simulink model "Tra_Add"  (R2016b)
settings: configuration reference "CodeGenConfigSet" (kept outside this file)
values from neighbouring files (symbols this model uses):
  Tra_bCanAirCanPtd_C = Calibration.Parameter    [init_Tra_Add.m]    (also in init_Tra_Add_SIL.m = Simulink.Parameter)
  Tra_bCanClntCanPtd_C = Calibration.Parameter    [init_Tra_Add.m]    (also in init_Tra_Add_SIL.m = Simulink.Parameter)
  Tra_rClgDem_C = Calibration.Parameter    [init_Tra_Add.m]    (also in init_Tra_Add_SIL.m = Simulink.Parameter)
  Tra_tClntDes_C = Calibration.Parameter    [init_Tra_Add.m]    (also in init_Tra_Add_SIL.m = Simulink.Parameter)
settings Model: Creator=Colin  LastModifiedBy=Colin
settings ConfigSetRef: SourceLocation=Base Workspace

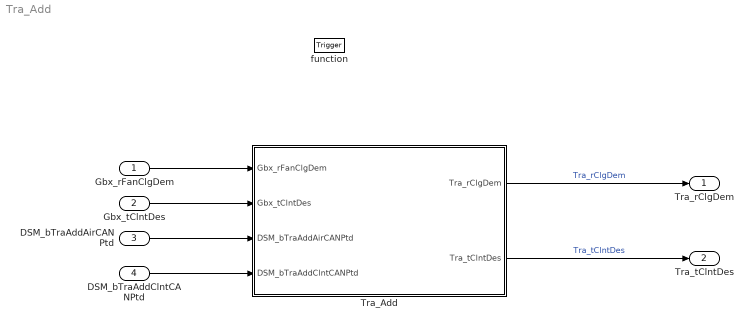
== system Tra_Add ==
  Gbx_rFanClgDem : Inport  Tag=%  Description=Percentage of fan cooling demand  OutMin=-300  OutMax=300  OutDataTypeStr=Prc_100_rate
  Gbx_tClntDes : Inport  Tag=deg  Description=Setpoint value of the coolant temperature (via CAN)  Port=2  OutMin=-150  OutMax=150  OutDataTypeStr=Temp_deg
  DSM_bTraAddAirCANPtd : Inport  Description=Function identifier relative cooling capacity over CAN  Port=3  OutMin=0  OutMax=1  OutDataTypeStr=boolean
  DSM_bTraAddClntCANPtd : Inport  Description=Function identifier set point value of the cooling capacity via CAN  Port=4  OutMin=0  OutMax=1  OutDataTypeStr=boolean
  function : TriggerPort  TriggerType=function-call  VariantControl=Variant
  Tra_Add : Subsystem
  Tra_rClgDem : Outport  Tag=%  Description=Relative fan cooling capacity  OutMin=-300  OutMax=300  OutDataTypeStr=Prc_100_rate
  Tra_tClntDes : Outport  Tag=deg  Description=Coolant temperature - Set point value  Port=2  OutMin=-150  OutMax=150  OutDataTypeStr=Temp_deg
  wires:
  Gbx_tClntDes/1 -> Tra_Add/2(Gbx_tClntDes)
  Gbx_rFanClgDem/1 -> Tra_Add/1(Gbx_rFanClgDem)
  DSM_bTraAddAirCANPtd/1 -> Tra_Add/3(DSM_bTraAddAirCANPtd)
  DSM_bTraAddClntCANPtd/1 -> Tra_Add/4(DSM_bTraAddClntCANPtd)
  Tra_Add/1(Tra_rClgDem) -> Tra_rClgDem/1  "Tra_rClgDem"
  Tra_Add/2(Tra_tClntDes) -> Tra_tClntDes/1  "Tra_tClntDes"

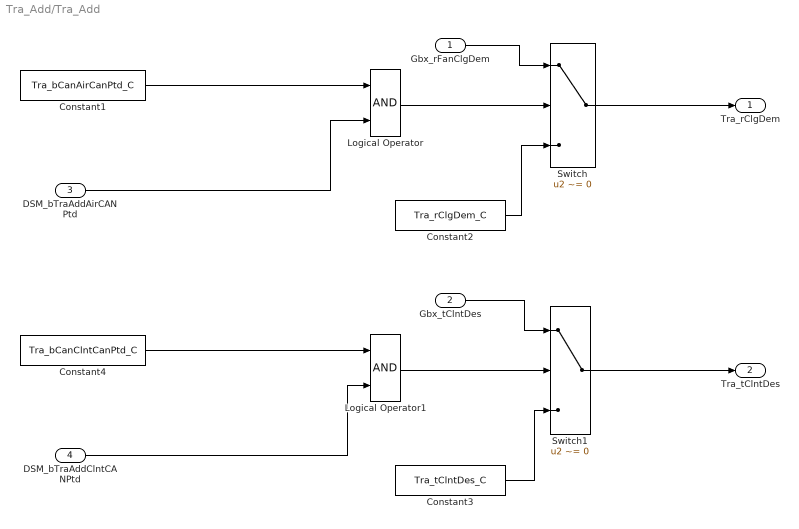
== system Tra_Add/Tra_Add ==
  Gbx_rFanClgDem : Inport  Tag=%%  Description=Percentage of fan cooling demand
  Gbx_tClntDes : Inport  Tag=deg  Description=Setpoint value of the coolant temperature (via CAN)  Port=2  OutMin=-150  OutMax=150  OutDataTypeStr=Temp_deg
  DSM_bTraAddAirCANPtd : Inport  Description=Function identifier relative cooling capacity over CAN  Port=3  OutMin=0  OutMax=1  OutDataTypeStr=boolean
  DSM_bTraAddClntCANPtd : Inport  Description=Function identifier set point value of the cooling capacity via CAN  Port=4  OutMin=0  OutMax=1  OutDataTypeStr=boolean
  Constant1 : Constant  Value=Tra_bCanAirCanPtd_C
  Constant2 : Constant  Value=Tra_rClgDem_C
  Constant3 : Constant  Value=Tra_tClntDes_C
  Constant4 : Constant  Value=Tra_bCanClntCanPtd_C
  Logical Operator : Logic  AllPortsSameDT=off  OutDataTypeStr=boolean
  Logical Operator1 : Logic  AllPortsSameDT=off  OutDataTypeStr=boolean
  Switch : Switch  Criteria=u2 ~= 0
  Switch1 : Switch  Criteria=u2 ~= 0
  Tra_rClgDem : Outport  Tag=%%  Description=Relative fan cooling capacity
  Tra_tClntDes : Outport  Tag=deg  Description=Coolant temperature - Set point value  Port=2  OutMin=-150  OutMax=150  OutDataTypeStr=Temp_deg
  wires:
  DSM_bTraAddAirCANPtd/1 -> Logical Operator/2
  Constant1/1 -> Logical Operator/1
  Logical Operator/1 -> Switch/2
  Constant2/1 -> Switch/3
  Gbx_rFanClgDem/1 -> Switch/1
  Switch/1 -> Tra_rClgDem/1
  DSM_bTraAddClntCANPtd/1 -> Logical Operator1/2
  Constant4/1 -> Logical Operator1/1
  Logical Operator1/1 -> Switch1/2
  Constant3/1 -> Switch1/3
  Gbx_tClntDes/1 -> Switch1/1
  Switch1/1 -> Tra_tClntDes/1
